simulink model "Afr"  (Simulink 8.4)
settings: Solver=ode45  StartTime=0.0  StopTime=10.0  RelTol=1e-3
undefined symbols (not defined in the file): Afr_facLambdaReqMan, Afr_facRatioMan, Afr_facStoich, Afr_flgLambdaReqOverride, Afr_flgRatioOverride
settings Model: Creator=YAL9FE  LastModifiedBy=ric9fe
settings DebuggingCC: FcnCallInpInsideContextMsg=EnableAllAsWarning

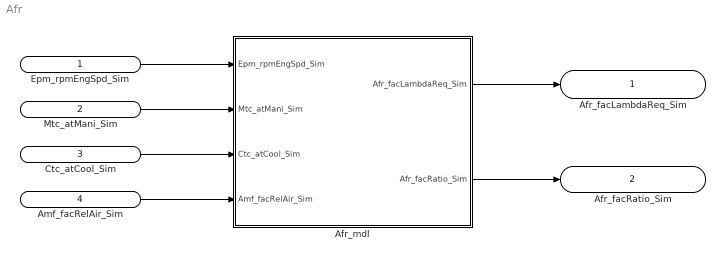
== system Afr ==
  Epm_rpmEngSpd_Sim : Inport
  Mtc_atMani_Sim : Inport  Port=2
  Ctc_atCool_Sim : Inport  Port=3
  Amf_facRelAir_Sim : Inport  Port=4
  Afr_mdl : Subsystem  mask(Functions){}
      mask help: AirFuelRatio
      mask Display:
      | image(imread('AirFuelRatio.jpg'))
      | port_label('input',1,'Epm_rpmEngSpd_Sim')
      | port_label('input',2,'Mtc_atMani_Sim')
      | port_label('input',3,'Ctc_atCool_Sim')
      | port_label('input',4,'Amf_facRelAir_Sim')
      | port_label('output',1,'Afr_facLambdaReq_Sim')
      | port_label('output',2,'Afr_facRatio_Sim')
  Afr_facLambdaReq_Sim : Outport
  Afr_facRatio_Sim : Outport  Port=2
  wires:
  Epm_rpmEngSpd_Sim/1 -> Afr_mdl/1(Epm_rpmEngSpd_Sim)
  Mtc_atMani_Sim/1 -> Afr_mdl/2(Mtc_atMani_Sim)
  Ctc_atCool_Sim/1 -> Afr_mdl/3(Ctc_atCool_Sim)
  Amf_facRelAir_Sim/1 -> Afr_mdl/4(Amf_facRelAir_Sim)
  Afr_mdl/1(Afr_facLambdaReq_Sim) -> Afr_facLambdaReq_Sim/1
  Afr_mdl/2(Afr_facRatio_Sim) -> Afr_facRatio_Sim/1

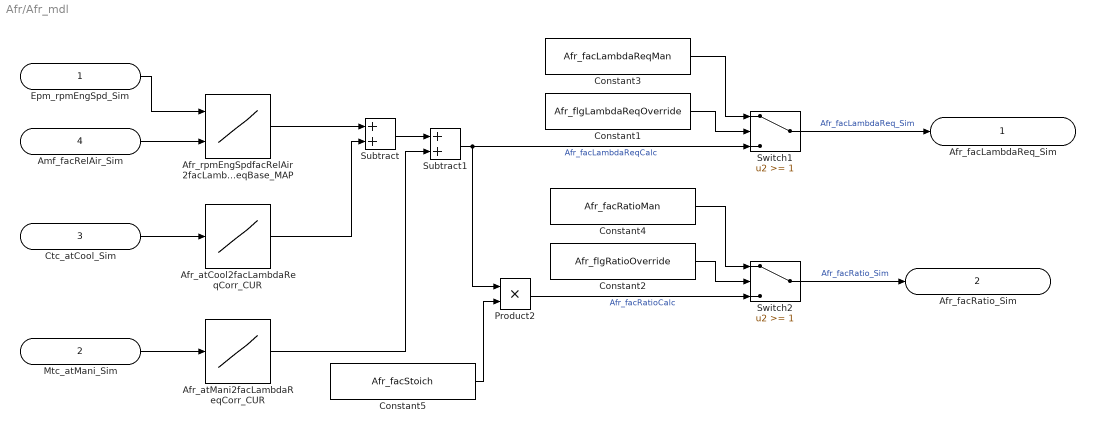
== system Afr/Afr_mdl ==
  Epm_rpmEngSpd_Sim : Inport
  Mtc_atMani_Sim : Inport  Port=2
  Ctc_atCool_Sim : Inport  Port=3
  Amf_facRelAir_Sim : Inport  Port=4
  Afr_atCool2facLambdaReqCorr_CUR : Lookup_n-D  NumberOfTableDimensions=1  BreakpointsForDimension1=[1:3]  Table=[4 5 6]  ExtrapMethod=Clip  InputSameDT=on
  Afr_atMani2facLambdaReqCorr_CUR : Lookup_n-D  NumberOfTableDimensions=1  BreakpointsForDimension1=[1:3]  Table=[4 5 6]  ExtrapMethod=Clip  InputSameDT=on
  Afr_rpmEngSpdfacRelAir2facLambdaReqBase_MAP : Lookup_n-D  BreakpointsForDimension1=[1:3]  BreakpointsForDimension2=[1:3]  ExtrapMethod=Clip  InputSameDT=on
  Constant1 : Constant  Value=Afr_flgLambdaReqOverride
  Constant2 : Constant  Value=Afr_flgRatioOverride
  Constant3 : Constant  Value=Afr_facLambdaReqMan
  Constant4 : Constant  Value=Afr_facRatioMan
  Constant5 : Constant  Value=Afr_facStoich
  Product2 : Product  OutDataTypeStr=Inherit: Same as first input
  Subtract : Sum  OutDataTypeStr=Inherit: Same as first input
  Subtract1 : Sum  OutDataTypeStr=Inherit: Same as first input
  Switch1 : Switch  Threshold=1
  Switch2 : Switch  Threshold=1
  Afr_facLambdaReq_Sim : Outport
  Afr_facRatio_Sim : Outport  Port=2
  wires:
  Epm_rpmEngSpd_Sim/1 -> Afr_rpmEngSpdfacRelAir2facLambdaReqBase_MAP/1
  Amf_facRelAir_Sim/1 -> Afr_rpmEngSpdfacRelAir2facLambdaReqBase_MAP/2
  Afr_rpmEngSpdfacRelAir2facLambdaReqBase_MAP/1 -> Subtract/1
  Subtract/1 -> Subtract1/1
  Ctc_atCool_Sim/1 -> Afr_atCool2facLambdaReqCorr_CUR/1
  Afr_atCool2facLambdaReqCorr_CUR/1 -> Subtract/2
  Mtc_atMani_Sim/1 -> Afr_atMani2facLambdaReqCorr_CUR/1
  Afr_atMani2facLambdaReqCorr_CUR/1 -> Subtract1/2
  Subtract1/1 -> Switch1/3, Product2/1  "Afr_facLambdaReqCalc"
  Constant1/1 -> Switch1/2
  Constant3/1 -> Switch1/1
  Switch1/1 -> Afr_facLambdaReq_Sim/1  "Afr_facLambdaReq_Sim"
  Switch2/1 -> Afr_facRatio_Sim/1  "Afr_facRatio_Sim"
  Product2/1 -> Switch2/3  "Afr_facRatioCalc"
  Constant5/1 -> Product2/2
  Constant2/1 -> Switch2/2
  Constant4/1 -> Switch2/1
